simulink model "IHC_NL_Logarithmic_Function_fil"  (R2019b)
settings: Solver=VariableStepAuto  StartTime=0.0  StopTime=testtime  RelTol=1e-3
InitFcn:
  | IHC_NL_Logarithmic_Test_Parameters
StopFcn:
  | Verify_IHC_NL_Logarithmic_Function_fil
values from neighbouring files (symbols this model uses):
  Fs = 48e3    (= 48000)    [IHC_NL_Logarithmic_Test_Parameters.m]
  ihcasym = 3.0    (= 3)    [IHC_NL_Logarithmic_Test_Parameters.m]
  slope = 0.1    [IHC_NL_Logarithmic_Test_Parameters.m]
  strength = (20.0e6)/(10^(corner/20))    (= 2000)    [IHC_NL_Logarithmic_Test_Parameters.m]
libraries: hdlmdlgenlib x2, dspsrcs4 x2, simulink x1, fillib x1
settings Model: Creator=mblun  LastModifiedBy=t96f346
settings OptimizationCC: BlockReduction=off  ConditionallyExecuteInputs=off  DefaultParameterBehavior=Inlined
settings DebuggingCC: AlgebraicLoopMsg=error  InheritedTsInSrcMsg=none
settings HardwareCC: ProdBitPerPointer=32  ProdBitPerSizeT=32  ProdBitPerPtrDiffT=32  ProdLargestAtomicFloat=None  ProdIntDivRoundTo=Undefined  ProdEndianess=Unspecified  ProdWordSize=32  ProdHWDeviceType=ASIC/FPGA->ASIC/FPGA  TargetBitPerPointer=64  TargetBitPerSizeT=64  TargetBitPerPtrDiffT=64  TargetLongLongMode=on  TargetIntDivRoundTo=Zero  TargetEndianess=LittleEndian  TargetWordSize=64  TargetHWDeviceType=Custom Processor->MATLAB Host Computer  ProdEqTarget=off
settings SFSimCC: CustomCodeUndefinedFunction=UseInterfaceOnly

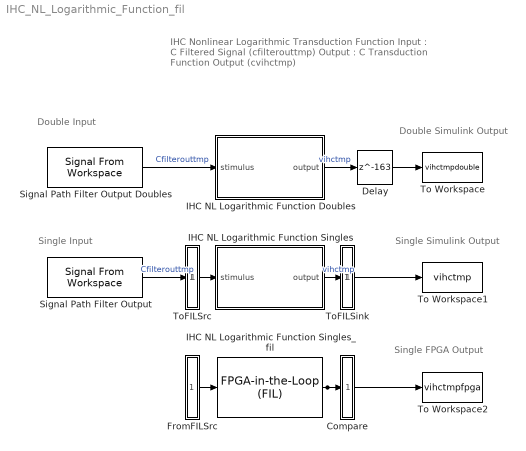
== system IHC_NL_Logarithmic_Function_fil ==
  note: IHC Nonlinear Logarithmic Transduction Function
      |
      | Input : C Filtered Signal (cfilterouttmp)
      |
      | Output : C Transduction Function Output (cvihctmp)
  note: Single Simulink Output
  note: Single FPGA Output
  note: Double Simulink Output
  note: Single Input
  note: Double Input
  Compare : Subsystem
      mask Display: disp('')
  Delay : Delay  DelayLength=163
  FromFILSrc : Subsystem
      mask Display: disp('')
  IHC NL Logarithmic Function Doubles : Subsystem
  IHC NL Logarithmic Function Singles : Subsystem
  IHC NL Logarithmic Function Singles_fil : fillib/FPGA-in-the-Loop (FIL)  ForceInterfaceUpdate=0.09754
      settings: SourceProductName=HDL Coder  SourceProductBaseCode=HD
  Signal Path Filter Output : dspsrcs4/Signal From Workspace  X=RxSignal  Ts=1/Fs  nsamps=1  OutputAfterFinalValue=Setting to zero  ignoreOrWarnInputAndFrameLengths=off  OutputFrames=off
  Signal Path Filter Output Doubles : dspsrcs4/Signal From Workspace  X=RxSignalDouble  Ts=1/Fs  nsamps=1  OutputAfterFinalValue=Setting to zero  ignoreOrWarnInputAndFrameLengths=off  OutputFrames=off
  To Workspace : ToWorkspace  VariableName=vihctmpdouble  SampleTime=-1
      settings: Save2DSignal=2-D array (concatenate along first dimension)
  To Workspace1 : ToWorkspace  VariableName=vihctmp  SampleTime=-1
      settings: Save2DSignal=2-D array (concatenate along first dimension)
  To Workspace2 : ToWorkspace  VariableName=vihctmpfpga  SampleTime=-1
      settings: Save2DSignal=2-D array (concatenate along first dimension)
  ToFILSink : Subsystem
      mask Display: disp('')
  ToFILSrc : Subsystem
      mask Display: disp('')
  wires:
  Signal Path Filter Output Doubles/1 -> IHC NL Logarithmic Function Doubles/1(stimulus)  "Cfilterouttmp"
  IHC NL Logarithmic Function Doubles/1(output) -> Delay/1  "vihctmp"
  ToFILSrc/1(out1) -> IHC NL Logarithmic Function Singles/1(stimulus)
  IHC NL Logarithmic Function Singles/1(output) -> ToFILSink/1(in1)  "vihctmp"
  Signal Path Filter Output/1 -> ToFILSrc/1(in1)  "Cfilterouttmp"
  ToFILSink/1(out1) -> To Workspace1/1
  FromFILSrc/1(out1) -> IHC NL Logarithmic Function Singles_fil/1
  IHC NL Logarithmic Function Singles_fil/1 -> To Workspace2/1, Compare/1(in1)
  Delay/1 -> To Workspace/1

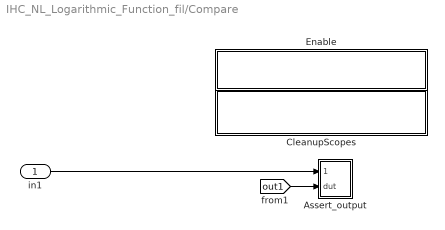
== system IHC_NL_Logarithmic_Function_fil/Compare ==
  in1 : Inport
  Assert_output : Subsystem  mask{ToleranceValue=1e-07}
  CleanupScopes : Subsystem
      settings: OpenFcn=|
      | blkName = gcb; %self block
      | idx = regexp(blkName, '/CleanupScopes$', 'once');
      | blkParent = blkName(1:idx-1);
      | blks=find_system(blkParent, 'LookUnderMasks', 'all','blocktype', 'Scope');
      | for itr = 1:length(blks)
      | 	 hScopeCfg = get_param(blks{itr},'ScopeConfiguration');
      | 	 hScopeCfg.Visible = ~ hScopeCfg.Visible;
      | end
      | drawnow;
      mask Display: fprintf(message('hdlcoder:cosim:vnl_dblclick').getString());
  Enable : Subsystem
      settings: OpenFcn=|
      | blkName = gcb;
      | idx = regexp(blkName, '/Enable$', 'once');
      | blkParent = blkName(1:idx-1);
      | blks=find_system(blkParent, 'LookUnderMasks', 'all','blocktype', 'Assertion');
      | e = get_param(blks{1}, 'Enabled');
      | if strcmp(e, 'on'), f= 'off';, else, f = 'on';, end
      | for ii=1:length(blks), set_param(blks{ii}, 'Enabled', f);, end
      | set_param(gcb, 'MaskDisplay',['fprintf(message(''hdlcoder:cosim:vnl_dblclick_assertions'',','''',upper(e),'''',').getString())']);
      mask Display: fprintf(message('hdlcoder:cosim:vnl_dblclick_assertions','OFF').getString());
  wires:
  in1/1 -> Assert_output/1(cosim)
  [out1] -> Assert_output/2(dut)

== system IHC_NL_Logarithmic_Function_fil/FromFILSrc ==
  dtc1 : DataTypeConversion  OutDataTypeStr=single  SaturateOnIntegerOverflow=on  RndMeth=Zero
  out1 : Outport
  wires:
  [in1] -> dtc1/1
  dtc1/1 -> out1/1

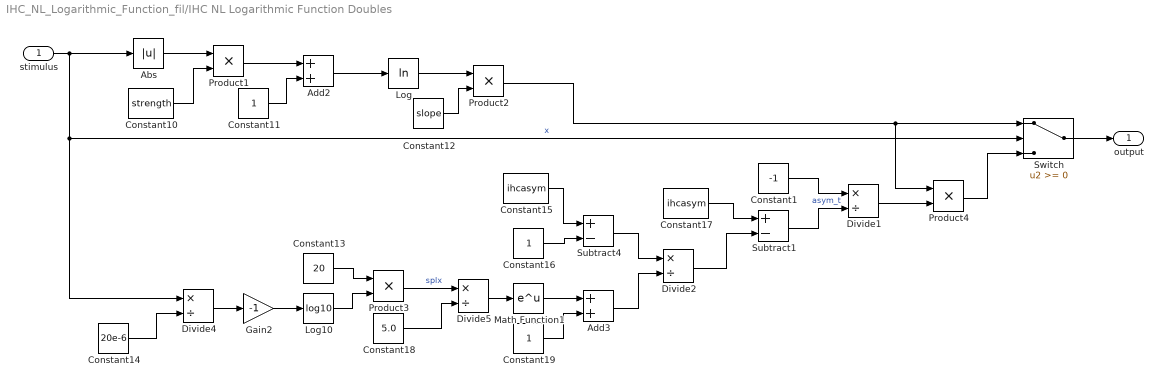
== system IHC_NL_Logarithmic_Function_fil/IHC NL Logarithmic Function Doubles ==
  stimulus : Inport
  Abs : Abs
  Add2 : Sum
  Add3 : Sum
  Constant1 : Constant  Value=-1  SampleTime=-1
  Constant10 : Constant  Value=strength  SampleTime=-1
  Constant11 : Constant  SampleTime=-1
  Constant12 : Constant  Value=slope  SampleTime=-1
  Constant13 : Constant  Value=20  SampleTime=-1
  Constant14 : Constant  Value=20e-6  SampleTime=-1
  Constant15 : Constant  Value=ihcasym  SampleTime=-1
  Constant16 : Constant  SampleTime=-1
  Constant17 : Constant  Value=ihcasym  SampleTime=-1
  Constant18 : Constant  Value=5.0  SampleTime=-1
  Constant19 : Constant  SampleTime=-1
  Divide{1..2,4..5} (4 alike) : Product  Inputs=*/  SaturateOnIntegerOverflow=on  RndMeth=Zero
  Gain2 : Gain  Gain=-1
  Log : Math  Operator=log  SaturateOnIntegerOverflow=on
  Log10 : Math  Operator=log10  SaturateOnIntegerOverflow=on
  Math Function1 : Math  SaturateOnIntegerOverflow=on
  Product{1..4} (4 alike) : Product
  Subtract1 : Sum  Inputs=+-
  Subtract4 : Sum  Inputs=+-
  Switch : Switch
  output : Outport  VectorParamsAs1DForOutWhenUnconnected=off
  wires:
  stimulus/1 -> Divide4/1, Switch/2, Abs/1  "x"
  Abs/1 -> Product1/1
  Constant10/1 -> Product1/2
  Constant11/1 -> Add2/2
  Product1/1 -> Add2/1
  Add2/1 -> Log/1
  Log/1 -> Product2/1
  Constant12/1 -> Product2/2
  Product2/1 -> Product4/1, Switch/1
  Constant14/1 -> Divide4/2
  Divide4/1 -> Gain2/1
  Gain2/1 -> Log10/1
  Log10/1 -> Product3/2
  Constant13/1 -> Product3/1
  Product3/1 -> Divide5/1  "splx"
  Constant15/1 -> Subtract4/1
  Constant16/1 -> Subtract4/2
  Constant18/1 -> Divide5/2
  Divide5/1 -> Math Function1/1
  Math Function1/1 -> Add3/1
  Constant19/1 -> Add3/2
  Subtract4/1 -> Divide2/1
  Add3/1 -> Divide2/2
  Constant17/1 -> Subtract1/1
  Divide2/1 -> Subtract1/2
  Subtract1/1 -> Divide1/2  "asym_t"
  Constant1/1 -> Divide1/1
  Divide1/1 -> Product4/2
  Product4/1 -> Switch/3
  Switch/1 -> output/1

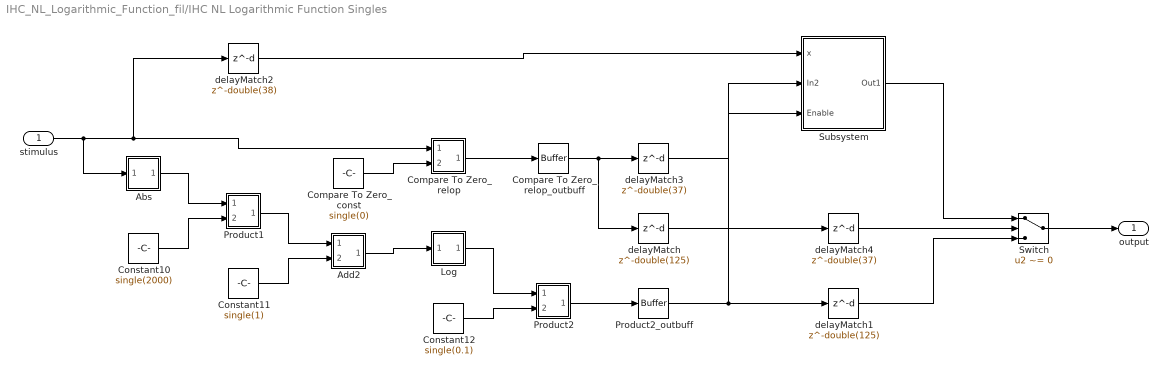
== system IHC_NL_Logarithmic_Function_fil/IHC NL Logarithmic Function Singles ==
  stimulus : Inport  OutDataTypeStr=single  PortDimensions=1  SampleTime=2.08333333333333e-05
  Abs : Subsystem
      mask Display: disp('NFP\nabs');
  Add2 : Subsystem
      mask Display: disp('NFP\nadd');
  Compare To Zero_const : Constant  Value=single(0)  OutDataTypeStr=single  SampleTime=-1
  Compare To Zero_relop : Subsystem
      mask Display: disp('NFP\nrelop');
  Compare To Zero_relop_outbuff : hdlmdlgenlib/Buffer
      settings: SourceProductName=Simulink  SourceProductBaseCode=SL
  Constant10 : Constant  Value=single(2000)  OutDataTypeStr=single  SampleTime=-1
  Constant11 : Constant  Value=single(1)  OutDataTypeStr=single  SampleTime=-1
  Constant12 : Constant  Value=single(0.1)  OutDataTypeStr=single  SampleTime=-1
  Log : Subsystem
      mask Display: disp('NFP\nmath');
  Product1 : Subsystem
      mask Display: disp('NFP\nmul');
  Product2 : Subsystem
      mask Display: disp('NFP\nmul');
  Product2_outbuff : hdlmdlgenlib/Buffer
      settings: SourceProductName=Simulink  SourceProductBaseCode=SL
  Subsystem : Subsystem
  Switch : Switch  Criteria=u2 ~= 0  Threshold=double(0)  OutDataTypeStr=single  SampleTime=2.08333333333333e-05
  delayMatch : Delay  DelayLength=double(125)  InitialCondition=0  SampleTime=2.08333333333333e-05
  delayMatch1 : Delay  DelayLength=double(125)  InitialCondition=0  SampleTime=2.08333333333333e-05
  delayMatch2 : Delay  DelayLength=double(38)  InitialCondition=0  SampleTime=2.08333333333333e-05
  delayMatch3 : Delay  DelayLength=double(37)  InitialCondition=0  SampleTime=2.08333333333333e-05
  delayMatch4 : Delay  DelayLength=double(37)  InitialCondition=0  SampleTime=2.08333333333333e-05
  output : Outport  VectorParamsAs1DForOutWhenUnconnected=off
  wires:
  delayMatch/1 -> delayMatch4/1
  Compare To Zero_relop_outbuff/1 -> delayMatch/1, delayMatch3/1
  stimulus/1 -> Compare To Zero_relop/1(In1), delayMatch2/1, Abs/1(In1)
  Product2/1(Out1) -> Product2_outbuff/1
  Product1/1(Out1) -> Add2/1(In1)
  Log/1(Out1) -> Product2/1(In1)
  Compare To Zero_relop/1(Out1) -> Compare To Zero_relop_outbuff/1
  Add2/1(Out1) -> Log/1(In1)
  Abs/1(Out1) -> Product1/1(In1)
  Product2_outbuff/1 -> Subsystem/2(In2), delayMatch1/1
  delayMatch3/1 -> Subsystem/3(Enable)
  Compare To Zero_const/1 -> Compare To Zero_relop/2(In2)
  Switch/1 -> output/1
  Subsystem/1(Out1) -> Switch/1
  delayMatch1/1 -> Switch/3
  Constant12/1 -> Product2/2(In2)
  Constant11/1 -> Add2/2(In2)
  Constant10/1 -> Product1/2(In2)
  delayMatch4/1 -> Switch/2
  delayMatch2/1 -> Subsystem/1(x)

== system IHC_NL_Logarithmic_Function_fil/ToFILSink ==
  in1 : Inport
  out1 : Outport
  tag scope: out1=global
  wires:
  in1/1 -> out1/1, [out1]

== system IHC_NL_Logarithmic_Function_fil/ToFILSrc ==
  in1 : Inport
  out1 : Outport
  tag scope: in1=global
  wires:
  in1/1 -> out1/1, [in1]

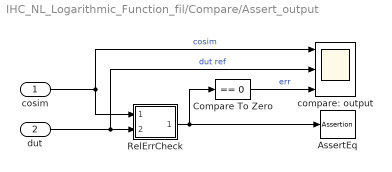
== system IHC_NL_Logarithmic_Function_fil/Compare/Assert_output ==
  cosim : Inport
  dut : Inport  Port=2
  AssertEq : Assertion  StopWhenAssertionFail=off
  Compare To Zero : simulink/Logic and Bit Operations/Compare To Zero  relop===  OutDataTypeStr=boolean
  RelErrCheck : Subsystem
  compare: output : Scope  NumInputPorts=3
  wires:
  dut/1 -> compare: output/2, RelErrCheck/2(In2)  "dut ref"
  cosim/1 -> compare: output/1, RelErrCheck/1(In1)  "cosim"
  RelErrCheck/1(Out1) -> AssertEq/1, Compare To Zero/1
  Compare To Zero/1 -> compare: output/3  "err"

== system IHC_NL_Logarithmic_Function_fil/Compare/CleanupScopes ==

== system IHC_NL_Logarithmic_Function_fil/Compare/Enable ==

== system IHC_NL_Logarithmic_Function_fil/IHC NL Logarithmic Function Singles/Abs ==
  In1 : Inport
  Abs : Abs  SampleTime=2.08333333333333e-05  OutDataTypeStr=single
  Out1 : Outport
  wires:
  Abs/1 -> Out1/1
  In1/1 -> Abs/1

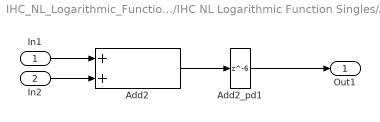
== system IHC_NL_Logarithmic_Function_fil/IHC NL Logarithmic Function Singles/Add2 ==
  In1 : Inport
  In2 : Inport  Port=2
  Add2 : Sum  OutDataTypeStr=single  SampleTime=2.08333333333333e-05  SaturateOnIntegerOverflow=on  InputSameDT=on
  Add2_pd1 : Delay  DelayLength=6
  Out1 : Outport
  wires:
  Add2_pd1/1 -> Out1/1
  Add2/1 -> Add2_pd1/1
  In2/1 -> Add2/2
  In1/1 -> Add2/1

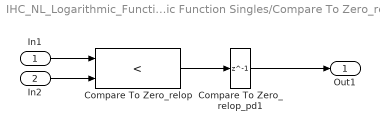
== system IHC_NL_Logarithmic_Function_fil/IHC NL Logarithmic Function Singles/Compare To Zero_relop ==
  In1 : Inport
  In2 : Inport  Port=2
  Compare To Zero_relop : RelationalOperator  Operator=<  OutDataTypeStr=boolean  SampleTime=2.08333333333333e-05  RndMeth=Nearest  InputSameDT=on
  Compare To Zero_relop_pd1 : Delay  DelayLength=1
  Out1 : Outport
  wires:
  Compare To Zero_relop_pd1/1 -> Out1/1
  Compare To Zero_relop/1 -> Compare To Zero_relop_pd1/1
  In2/1 -> Compare To Zero_relop/2
  In1/1 -> Compare To Zero_relop/1

== system IHC_NL_Logarithmic_Function_fil/IHC NL Logarithmic Function Singles/Log ==
  In1 : Inport
  Log : Math  Operator=log  SampleTime=2.08333333333333e-05  SaturateOnIntegerOverflow=on
  Log_pd1 : Delay  DelayLength=20
  Out1 : Outport
  wires:
  Log_pd1/1 -> Out1/1
  Log/1 -> Log_pd1/1
  In1/1 -> Log/1

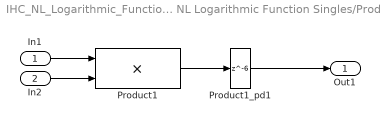
== system IHC_NL_Logarithmic_Function_fil/IHC NL Logarithmic Function Singles/Product1 ==
  In1 : Inport
  In2 : Inport  Port=2
  Product1 : Product  Inputs=**  OutDataTypeStr=single  SampleTime=2.08333333333333e-05
  Product1_pd1 : Delay  DelayLength=6
  Out1 : Outport
  wires:
  Product1_pd1/1 -> Out1/1
  Product1/1 -> Product1_pd1/1
  In2/1 -> Product1/2
  In1/1 -> Product1/1

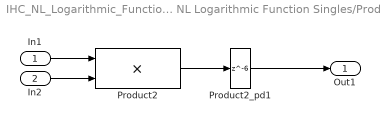
== system IHC_NL_Logarithmic_Function_fil/IHC NL Logarithmic Function Singles/Product2 ==
  In1 : Inport
  In2 : Inport  Port=2
  Product2 : Product  Inputs=**  OutDataTypeStr=single  SampleTime=2.08333333333333e-05
  Product2_pd1 : Delay  DelayLength=6
  Out1 : Outport
  wires:
  Product2_pd1/1 -> Out1/1
  Product2/1 -> Product2_pd1/1
  In2/1 -> Product2/2
  In1/1 -> Product2/1

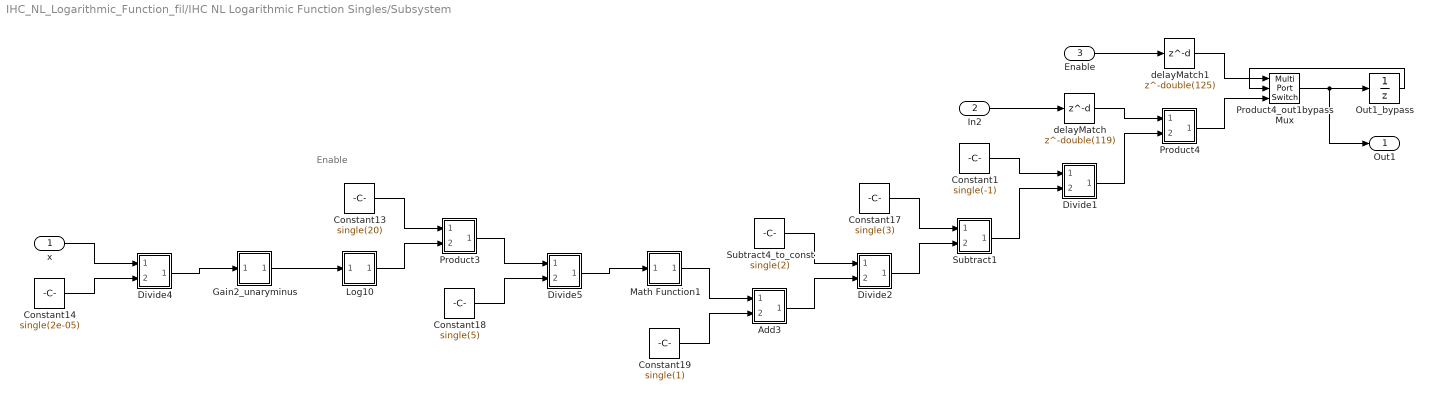
== system IHC_NL_Logarithmic_Function_fil/IHC NL Logarithmic Function Singles/Subsystem ==
  note: Enable
  x : Inport  OutDataTypeStr=single  PortDimensions=1  SampleTime=2.08333333333333e-05
  In2 : Inport  Port=2  OutDataTypeStr=single  PortDimensions=1  SampleTime=2.08333333333333e-05
  Enable : Inport  Port=3  OutDataTypeStr=boolean  SampleTime=2.08333333333333e-05
  Add3 : Subsystem
      mask Display: disp('NFP\nadd');
  Constant1 : Constant  Value=single(-1)  OutDataTypeStr=single  SampleTime=-1
  Constant13 : Constant  Value=single(20)  OutDataTypeStr=single  SampleTime=-1
  Constant14 : Constant  Value=single(2e-05)  OutDataTypeStr=single  SampleTime=-1
  Constant17 : Constant  Value=single(3)  OutDataTypeStr=single  SampleTime=-1
  Constant18 : Constant  Value=single(5)  OutDataTypeStr=single  SampleTime=-1
  Constant19 : Constant  Value=single(1)  OutDataTypeStr=single  SampleTime=-1
  Divide1 : Subsystem
      mask Display: disp('NFP\nmul');
  Divide2 : Subsystem
      mask Display: disp('NFP\nmul');
  Divide4 : Subsystem
      mask Display: disp('NFP\nmul');
  Divide5 : Subsystem
      mask Display: disp('NFP\nmul');
  Gain2_unaryminus : Subsystem
      mask Display: disp('NFP\numinus');
  Log10 : Subsystem
      mask Display: disp('NFP\nmath');
  Math Function1 : Subsystem
      mask Display: disp('NFP\nmath');
  Out1_bypass : UnitDelay  SampleTime=2.08333333333333e-05
  Product3 : Subsystem
      mask Display: disp('NFP\nmul');
  Product4 : Subsystem
      mask Display: disp('NFP\nmul');
  Product4_out1bypassMux : MultiPortSwitch  DataPortOrder=Zero-based contiguous  Inputs=2  zeroidx=on  OutDataTypeStr=single  SampleTime=2.08333333333333e-05
  Subtract1 : Subsystem
      mask Display: disp('NFP\nadd');
  Subtract4_to_const : Constant  Value=single(2)  OutDataTypeStr=single  SampleTime=-1
  delayMatch : Delay  DelayLength=double(119)  InitialCondition=0
  delayMatch1 : Delay  DelayLength=double(125)  InitialCondition=0
  Out1 : Outport  OutDataTypeStr=single  InitialOutput=0
  wires:
  Out1_bypass/1 -> Product4_out1bypassMux/2
  Enable/1 -> delayMatch1/1
  In2/1 -> delayMatch/1
  x/1 -> Divide4/1(In1)
  Product4_out1bypassMux/1 -> Out1_bypass/1, Out1/1
  Subtract1/1(Out1) -> Divide1/2(In2)
  Product4/1(Out1) -> Product4_out1bypassMux/3
  Product3/1(Out1) -> Divide5/1(In1)
  Math Function1/1(Out1) -> Add3/1(In1)
  Log10/1(Out1) -> Product3/2(In2)
  Divide5/1(Out1) -> Math Function1/1(In1)
  Divide4/1(Out1) -> Gain2_unaryminus/1(In1)
  Divide2/1(Out1) -> Subtract1/2(In2)
  Divide1/1(Out1) -> Product4/2(In2)
  Add3/1(Out1) -> Divide2/2(In2)
  Gain2_unaryminus/1(Out1) -> Log10/1(In1)
  Subtract4_to_const/1 -> Divide2/1(In1)
  Constant19/1 -> Add3/2(In2)
  Constant18/1 -> Divide5/2(In2)
  Constant17/1 -> Subtract1/1(In1)
  Constant14/1 -> Divide4/2(In2)
  Constant13/1 -> Product3/1(In1)
  Constant1/1 -> Divide1/1(In1)
  delayMatch/1 -> Product4/1(In1)
  delayMatch1/1 -> Product4_out1bypassMux/1

== system IHC_NL_Logarithmic_Function_fil/Compare/Assert_output/RelErrCheck ==
  In1 : Inport
  In2 : Inport  Port=2
  "RelativeErrorCheck " : MATLAB Function  TreatAsAtomicUnit=on
  Out1 : Outport  VectorParamsAs1DForOutWhenUnconnected=off
  wires:
  In2/1 -> "RelativeErrorCheck "/2(R)
  In1/1 -> "RelativeErrorCheck "/1(P)
  "RelativeErrorCheck "/1(y) -> Out1/1

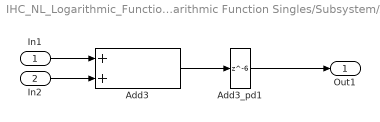
== system IHC_NL_Logarithmic_Function_fil/IHC NL Logarithmic Function Singles/Subsystem/Add3 ==
  In1 : Inport
  In2 : Inport  Port=2
  Add3 : Sum  OutDataTypeStr=single  SampleTime=2.08333333333333e-05  SaturateOnIntegerOverflow=on  InputSameDT=on
  Add3_pd1 : Delay  DelayLength=6
  Out1 : Outport
  wires:
  Add3_pd1/1 -> Out1/1
  Add3/1 -> Add3_pd1/1
  In2/1 -> Add3/2
  In1/1 -> Add3/1

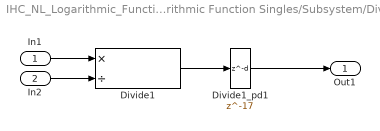
== system IHC_NL_Logarithmic_Function_fil/IHC NL Logarithmic Function Singles/Subsystem/Divide1 ==
  In1 : Inport
  In2 : Inport  Port=2
  Divide1 : Product  Inputs=*/  OutDataTypeStr=single  SampleTime=2.08333333333333e-05  SaturateOnIntegerOverflow=on  RndMeth=Zero
  Divide1_pd1 : Delay  DelayLength=17
  Out1 : Outport
  wires:
  Divide1_pd1/1 -> Out1/1
  Divide1/1 -> Divide1_pd1/1
  In2/1 -> Divide1/2
  In1/1 -> Divide1/1

== system IHC_NL_Logarithmic_Function_fil/IHC NL Logarithmic Function Singles/Subsystem/Divide2 ==
  In1 : Inport
  In2 : Inport  Port=2
  Divide2 : Product  Inputs=*/  OutDataTypeStr=single  SampleTime=2.08333333333333e-05  SaturateOnIntegerOverflow=on  RndMeth=Zero
  Divide2_pd1 : Delay  DelayLength=17
  Out1 : Outport
  wires:
  Divide2_pd1/1 -> Out1/1
  Divide2/1 -> Divide2_pd1/1
  In2/1 -> Divide2/2
  In1/1 -> Divide2/1

== system IHC_NL_Logarithmic_Function_fil/IHC NL Logarithmic Function Singles/Subsystem/Divide4 ==
  In1 : Inport
  In2 : Inport  Port=2
  Divide4 : Product  Inputs=*/  OutDataTypeStr=single  SampleTime=2.08333333333333e-05  SaturateOnIntegerOverflow=on  RndMeth=Zero
  Divide4_pd1 : Delay  DelayLength=17
  Out1 : Outport
  wires:
  Divide4_pd1/1 -> Out1/1
  Divide4/1 -> Divide4_pd1/1
  In2/1 -> Divide4/2
  In1/1 -> Divide4/1

== system IHC_NL_Logarithmic_Function_fil/IHC NL Logarithmic Function Singles/Subsystem/Divide5 ==
  In1 : Inport
  In2 : Inport  Port=2
  Divide5 : Product  Inputs=*/  OutDataTypeStr=single  SampleTime=2.08333333333333e-05  SaturateOnIntegerOverflow=on  RndMeth=Zero
  Divide5_pd1 : Delay  DelayLength=17
  Out1 : Outport
  wires:
  Divide5_pd1/1 -> Out1/1
  Divide5/1 -> Divide5_pd1/1
  In2/1 -> Divide5/2
  In1/1 -> Divide5/1

== system IHC_NL_Logarithmic_Function_fil/IHC NL Logarithmic Function Singles/Subsystem/Gain2_unaryminus ==
  In1 : Inport
  Gain2_unaryminus : UnaryMinus  SampleTime=2.08333333333333e-05
  Out1 : Outport
  wires:
  Gain2_unaryminus/1 -> Out1/1
  In1/1 -> Gain2_unaryminus/1

== system IHC_NL_Logarithmic_Function_fil/IHC NL Logarithmic Function Singles/Subsystem/Log10 ==
  In1 : Inport
  Log10 : Math  Operator=log10  SampleTime=2.08333333333333e-05  SaturateOnIntegerOverflow=on
  Log10_pd1 : Delay  DelayLength=17
  Out1 : Outport
  wires:
  Log10_pd1/1 -> Out1/1
  Log10/1 -> Log10_pd1/1
  In1/1 -> Log10/1

== system IHC_NL_Logarithmic_Function_fil/IHC NL Logarithmic Function Singles/Subsystem/Math Function1 ==
  In1 : Inport
  Math Function1 : Math  SampleTime=2.08333333333333e-05  SaturateOnIntegerOverflow=on
  Math Function1_pd1 : Delay  DelayLength=16
  Out1 : Outport
  wires:
  Math Function1_pd1/1 -> Out1/1
  Math Function1/1 -> Math Function1_pd1/1
  In1/1 -> Math Function1/1

== system IHC_NL_Logarithmic_Function_fil/IHC NL Logarithmic Function Singles/Subsystem/Product3 ==
  In1 : Inport
  In2 : Inport  Port=2
  Product3 : Product  Inputs=**  OutDataTypeStr=single  SampleTime=2.08333333333333e-05
  Product3_pd1 : Delay  DelayLength=6
  Out1 : Outport
  wires:
  Product3_pd1/1 -> Out1/1
  Product3/1 -> Product3_pd1/1
  In2/1 -> Product3/2
  In1/1 -> Product3/1

== system IHC_NL_Logarithmic_Function_fil/IHC NL Logarithmic Function Singles/Subsystem/Product4 ==
  In1 : Inport
  In2 : Inport  Port=2
  Product4 : Product  Inputs=**  OutDataTypeStr=single  SampleTime=2.08333333333333e-05
  Product4_pd1 : Delay  DelayLength=6
  Out1 : Outport
  wires:
  Product4_pd1/1 -> Out1/1
  Product4/1 -> Product4_pd1/1
  In2/1 -> Product4/2
  In1/1 -> Product4/1

== system IHC_NL_Logarithmic_Function_fil/IHC NL Logarithmic Function Singles/Subsystem/Subtract1 ==
  In1 : Inport
  In2 : Inport  Port=2
  Subtract1 : Sum  Inputs=+-  OutDataTypeStr=single  SampleTime=2.08333333333333e-05  SaturateOnIntegerOverflow=on  InputSameDT=on
  Subtract1_pd1 : Delay  DelayLength=6
  Out1 : Outport
  wires:
  Subtract1_pd1/1 -> Out1/1
  Subtract1/1 -> Subtract1_pd1/1
  In2/1 -> Subtract1/2
  In1/1 -> Subtract1/1

== matlab function IHC_NL_Logarithmic_Function_fil/Compare/Assert_output/RelErrCheck/RelativeErrorCheck  ==
  data: P input; y output; R input; ToleranceValue parameter double
% Check if the relative error of R with respect to P is below
% ToleranceValue
% P, R are floating-point
function y = relErrCheck(P,R, ToleranceValue)
    tol = ToleranceValue;
    sz = numel(P);
    assert(sz == numel(R), 'Inputs P and R have different sizes.');
    y = false(1, sz);

    for ii=1:sz
        if (isnan(P(ii)) || isnan(R(ii)))
            if (isnan(P(ii)) && isnan(R(ii)))
                y(ii) = true;
            end
        elseif (isinf(P(ii)) || isinf(R(ii)))
            y(ii) = (P(ii) == R(ii));
        elseif (P(ii) == 0)
            y(ii) = (R(ii) == 0);
        else
            absdiff = abs(P(ii) - R(ii));
            relerr = absdiff/abs(P(ii));
            y(ii) = (relerr <= tol);
        end
    end
end
